simulink model "motor_healthy"  (R2025a)
settings: Solver=FixedStepAuto  StartTime=0  StopTime=5  FixedStep=1e-4  RelTol=1e-3
model workspace (MAT data in the model file):
  Vin = 15
undefined symbols (not defined in the file): f_supply, Torque_in, V_in
libraries: spsAsynchronousMachineSIUnitsLib x1, spsThreePhaseSourceLib x1, sps_lib x1
settings Model: Creator=User  LastModifiedBy=User
settings DataIOCC: SaveOutput=off  DSMLogging=off  ReturnWorkspaceOutputs=off

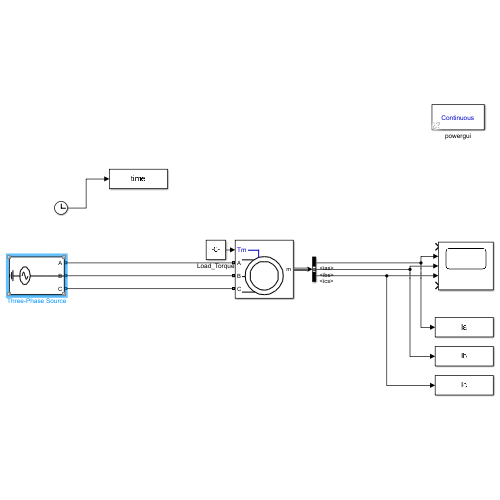
[thumbnail: Simulink's stored preview of the top-level diagram]
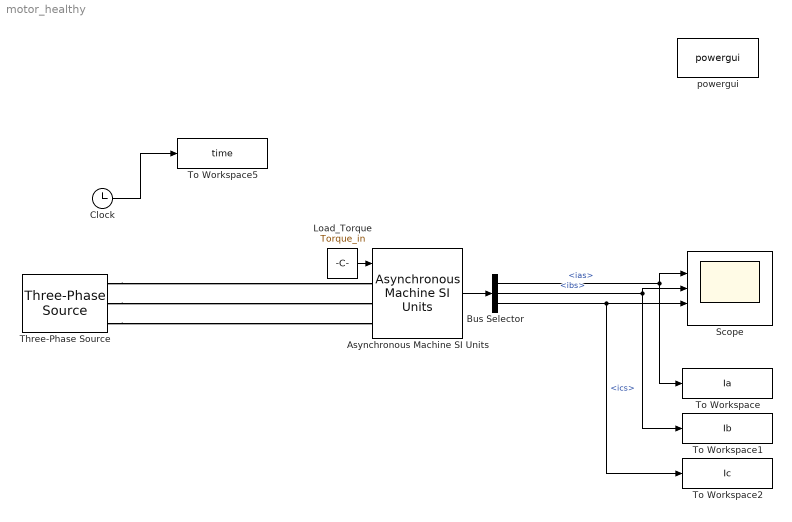
== system motor_healthy ==
  Asynchronous Machine SI Units : spsAsynchronousMachineSIUnitsLib/Asynchronous Machine SI Units  RotorType=Squirrel-cage  PresetModel=No  MechanicalLoad=Torque Tm  ShowDetailedParameters=on  ReferenceFrame=Stationary  Units=SI  MeasurementBus=on  NominalParameters=[7500 400 50]  VoltageRatio=1  Stator=[1.405 0.005839]  Rotor=[1.395 0.005839]  Cage1=[0.4155 0.002066]  Cage2=[0.4168 0.0003495]  Lm=0.1722  Mechanical=[0.0131 0.001 2]  PolePairs=2  InitialConditions=[0 0 0 0 0 0 0 0]  SimulateSaturation=off  Saturation=[14.03593122, 27.81365428, 53.79336849, 72.68890987, 97.98006896, 148.6815601, 215.7428561, 302.9841135, 428.7778367 ; 230, 322, 414, 460, 506, 552, 598, 644, 690]  LoadFlowParameters=1492000  TsPowergui=0  TsBlock=-1  IterativeModel=Trapezoidal non iterative  IterativeDiscreteModel=Trapezoidal non iterative  Pmec=1.492e+006
  Bus Selector : BusSelector  OutputSignals=ias,ibs,ics
  Clock : Clock
  Load_Torque : Constant  Value=Torque_in
  Scope : Scope  NumInputPorts=5
      settings: ActiveDisplayYMinimum=-1  ActiveDisplayYMaximum=1
  Three-Phase Source : spsThreePhaseSourceLib/Three-Phase Source  InternalConnection=Yg  VoltagePhases=on  Voltage=400  PhaseAngle=0  Voltage_phases=[V_in V_in V_in]/sqrt(3)  PhaseAngles_phases=[0 -120 +120]  Frequency=f_supply  NonIdealSource=off  SpecifyImpedance=off  Resistance=0.8929  Inductance=16.58e-3  ShortCircuitLevel=100e6  BaseVoltage=25e3  XRratio=7  BusType=swing  Pref=10e3  Qref=0  Prefabc=[10e3, 10e3, 10e3]  Qrefabc=[0, 0, 0]  Qmin=-inf  Qmax=inf
  To Workspace : ToWorkspace  VariableName=Ia  SampleTime=-1
  To Workspace1 : ToWorkspace  VariableName=Ib  SampleTime=-1
  To Workspace2 : ToWorkspace  VariableName=Ic  SampleTime=-1
  To Workspace5 : ToWorkspace  VariableName=time  SampleTime=-1
  powergui : sps_lib/powergui  Priority=1  SimulationMode=Continuous  SampleTime=50e-6  frequency=60  Iterations=50  frequencyindice=50  Pbase=100e6  ErrMax=1e-4  UnitsV=kV  UnitsW=MW  buscounter=0  FunctionMessages=off  echomessages=off  EnableUseOfTLC=off  CurrentSourceSwitches=off  DisableSnubberDevices=off  DisableRonSwitches=off  DisableVfSwitches=off  DisplayEquations=off  AutomaticDiscreteSolvers=off  SolverType=Tustin/Backward Euler (TBE)  Interpol=off  ExternalGateDelay=off  methode=off  Ts=100  x0status=blocks  SPID=on  SwTol=0  HookPort=off  NonlinearTolerance=1e-4  nMaxIteration=100  ContinueOnMaxIteration=off  RestoreLinks=warning  ResistiveCurrentMeasurement=off  Frange=[0:2:500]  Ylog=off  Xlog=on  ShowGrid=off  save=off  variable=ZData  structure=0  ZoomFFT=off  StartTime=0.0  cycles=1  DisplayStyle=1  fundamental=60  FreqAxis=off  MaxFrequency=1000  frequencyindicesteady=1  RmsSteady=1  display=off
  wires:
  Load_Torque/1 -> Asynchronous Machine SI Units/1
  Asynchronous Machine SI Units/1 -> Bus Selector/1
  Clock/1 -> To Workspace5/1
  Bus Selector/1 -> Scope/2, To Workspace/1  "<ias>"
  Bus Selector/2 -> To Workspace1/1, Scope/3  "<ibs>"
  Bus Selector/3 -> To Workspace2/1, Scope/4  "<ics>"
  connections:
  Three-Phase Source/RConn1 -- Asynchronous Machine SI Units/LConn1
  Three-Phase Source/RConn2 -- Asynchronous Machine SI Units/LConn2
  Three-Phase Source/RConn3 -- Asynchronous Machine SI Units/LConn3
